simulink model "Joey_Control"  (R2022b)
settings: Solver=VariableStepAuto  StartTime=0.0  StopTime=3  RelTol=1e-3
libraries: simulink_extras x4
settings Model: Creator=khemwutapornpipatsakul  LastModifiedBy=khemwutapornpipatsakul

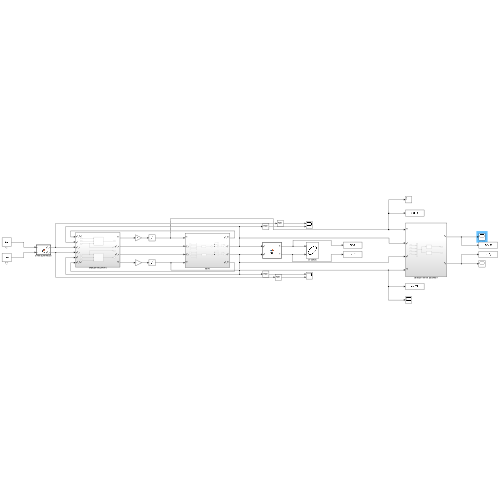
[thumbnail: Simulink's stored preview of the top-level diagram]
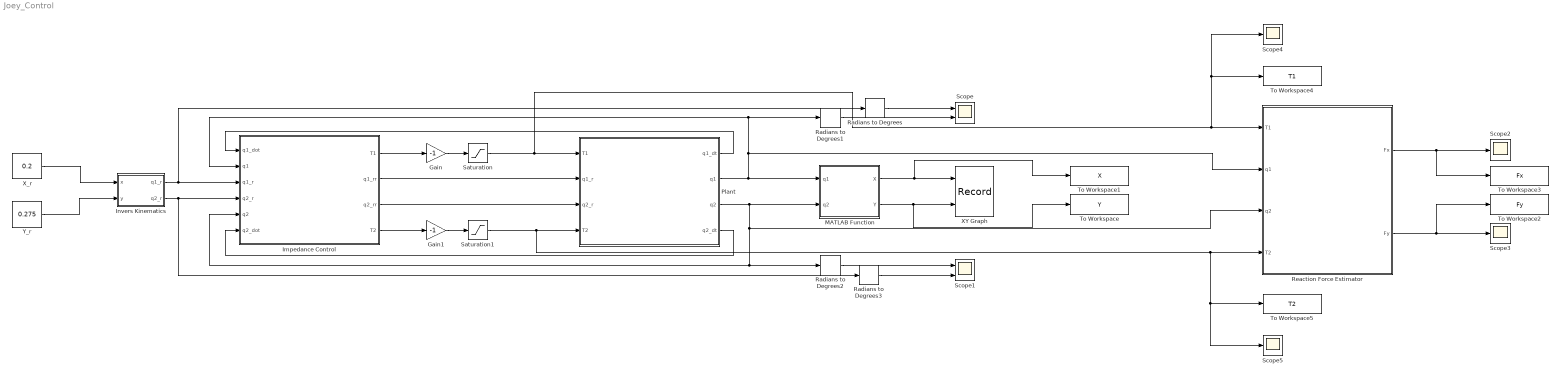
== system Joey_Control ==
  Gain : Gain  Gain=-1
  Gain1 : Gain  Gain=-1
  Impedance Control : Subsystem
  Invers Kinematics : MATLAB Function  TreatAsAtomicUnit=on
  MATLAB Function : MATLAB Function  TreatAsAtomicUnit=on
  Plant : Subsystem
  Radians to Degrees{,1..3} (4 alike) : simulink_extras/Transformations/Radians to Degrees
  Reaction Force Estimator : Subsystem
  Saturation : Saturate  UpperLimit=2  LowerLimit=-2
  Saturation1 : Saturate  UpperLimit=2  LowerLimit=-2
  Scope : Scope  NumInputPorts=2
  Scope1 : Scope  NumInputPorts=2
  Scope{2..5} (4 alike) : Scope
  To Workspace : ToWorkspace  VariableName=Y  SaveFormat=Timeseries  SampleTime=-1
  To Workspace1 : ToWorkspace  VariableName=X  SaveFormat=Timeseries  SampleTime=-1
  To Workspace2 : ToWorkspace  VariableName=Fy  SaveFormat=Timeseries  SampleTime=-1
  To Workspace3 : ToWorkspace  VariableName=Fx  SaveFormat=Timeseries  SampleTime=-1
  To Workspace4 : ToWorkspace  VariableName=T1  SaveFormat=Timeseries  SampleTime=-1
  To Workspace5 : ToWorkspace  VariableName=T2  SaveFormat=Timeseries  SampleTime=-1
  XY Graph : Record  FileSettingsInternal="{\"entries\":[{\"content\":{\"excelSettings\":{\"content\":{},\"type\":\"Streamout.ExcelSettings\"}},\"type\":\"Streamout.FileSettingStorage\",\"uuid\":\"b0abfdfa-5850-41cf-a1e0-bf550fd7b288\"}],\"packageUris\":[\"http://schema.mathworks.com/mf0/streamout_blocks/R2020a\"],\"version\":\"1.0\"}"  Layout=[1 1]  SignalsInternal="{\"entries\":[{\"content\":{\"signals\":[{\"content\":{\"blockPath\":[\"Joey_Control/XY Graph\"],\"channel\":[],\"dimensions\":[1],\"domain\":\"Joey_Control/XY Graph\",\"lineColor\":\"#a2142f\",\"plots\":[1],\"port\":1,\"sid\":[\"\"],\"signalID\":89,\"signalName\":\"MATLAB Function:1\"},\"type\":\"RecordBlkView.Signal\",\"uuid\":\"3823b3a6-9026-4afb-b3d4-39afb66ecd92\"},{\"content\":{\"blockPath\":[\"Joey_Control/XY Graph\"],\"channel\":[],\"dimensions\":[1],\"domain\":\"Joey_Control/XY Graph\",\"lineColor\":\"#139fff\",\"plots\":[1],\"port\":2,\"sid\":[\"\"],\"signalID\":93,\"signalName\":\"MATLAB Function:2\"},\"type\":\"RecordBlkView.Signal\",\"uuid\":\"4a1dff9e-01f1-4793-a448-94da4f18f44a\"}]},\"type\":\"RecordBlkView.InputSignals\",\"uuid\":\"29e68c19-1a98-4a03-81c8-2dcea01dd2a8\"}],\"packageUris\":[\"http://schema.mathworks.com/mf0/streamout_blocks/R2020a\"],\"version\":\"1.0\"}"  VisualizationBindings="{\"xyplotplugin\":{\"info\":[{\"series\":[{\"bindingParametersList\":[{\"parameter\":\"X-Axis\",\"signalID\":89,\"signalName\":\"MATLAB Function:1\"},{\"parameter\":\"Y-Axis\",\"signalID\":93,\"signalName\":\"MATLAB Function:2\"}],\"seriesID\":54391}],\"subplotID\":1}]}}"  CompatibilityTag=XY
  X_r : Constant  Value=0.2  SampleTime=0.01
  Y_r : Constant  Value=0.275  SampleTime=0.01
  wires:
  X_r/1 -> Invers Kinematics/1(x)
  Y_r/1 -> Invers Kinematics/2(y)
  Invers Kinematics/1(q1_r) -> Radians to Degrees/1, Impedance Control/3(q1_r)
  Invers Kinematics/2(q2_r) -> Radians to Degrees3/1, Impedance Control/4(q2_r)
  Impedance Control/1(T1) -> Gain/1
  Impedance Control/4(T2) -> Gain1/1
  Saturation/1 -> Scope4/1, To Workspace4/1, Reaction Force Estimator/1(T1), Plant/1(T1)
  Saturation1/1 -> Plant/4(T2), Scope5/1, To Workspace5/1, Reaction Force Estimator/4(T2)
  Impedance Control/2(q1_rr) -> Plant/2(q1_r)
  Impedance Control/3(q2_rr) -> Plant/3(q2_r)
  Plant/4(q2_dt) -> Impedance Control/6(q2_dot)
  Plant/1(q1_dt) -> Impedance Control/1(q1_dot)
  Plant/2(q1) -> MATLAB Function/1(q1), Impedance Control/2(q1), Radians to Degrees1/1, Reaction Force Estimator/2(q1)
  Plant/3(q2) -> Impedance Control/5(q2), Radians to Degrees2/1, Reaction Force Estimator/3(q2), MATLAB Function/2(q2)
  Gain/1 -> Saturation/1
  Gain1/1 -> Saturation1/1
  Reaction Force Estimator/1(Fx) -> To Workspace3/1, Scope2/1
  Reaction Force Estimator/2(Fy) -> To Workspace2/1, Scope3/1
  MATLAB Function/1(X) -> XY Graph/1, To Workspace1/1
  MATLAB Function/2(Y) -> XY Graph/2, To Workspace/1
  Radians to Degrees/1 -> Scope/1
  Radians to Degrees1/1 -> Scope/2
  Radians to Degrees2/1 -> Scope1/1
  Radians to Degrees3/1 -> Scope1/2

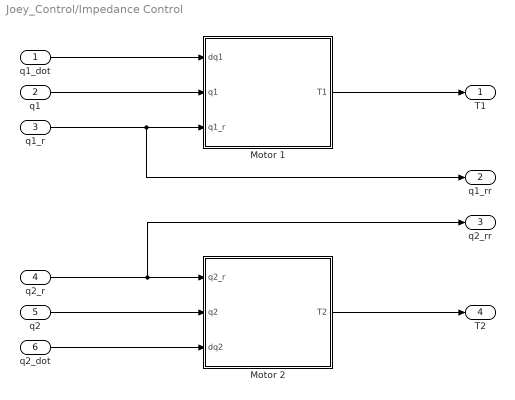
== system Joey_Control/Impedance Control ==
  q1_dot : Inport
  q1 : Inport  Port=2
  q1_r : Inport  Port=3
  q2_r : Inport  Port=4
  q2 : Inport  Port=5
  q2_dot : Inport  Port=6
  Motor 1 : MATLAB Function  TreatAsAtomicUnit=on
  Motor 2 : MATLAB Function  TreatAsAtomicUnit=on
  T1 : Outport
  q1_rr : Outport  Port=2
  q2_rr : Outport  Port=3
  T2 : Outport  Port=4
  wires:
  q1_dot/1 -> Motor 1/1(dq1)
  q1/1 -> Motor 1/2(q1)
  q1_r/1 -> q1_rr/1, Motor 1/3(q1_r)
  Motor 1/1(T1) -> T1/1
  q2_r/1 -> q2_rr/1, Motor 2/1(q2_r)
  q2/1 -> Motor 2/2(q2)
  q2_dot/1 -> Motor 2/3(dq2)
  Motor 2/1(T2) -> T2/1

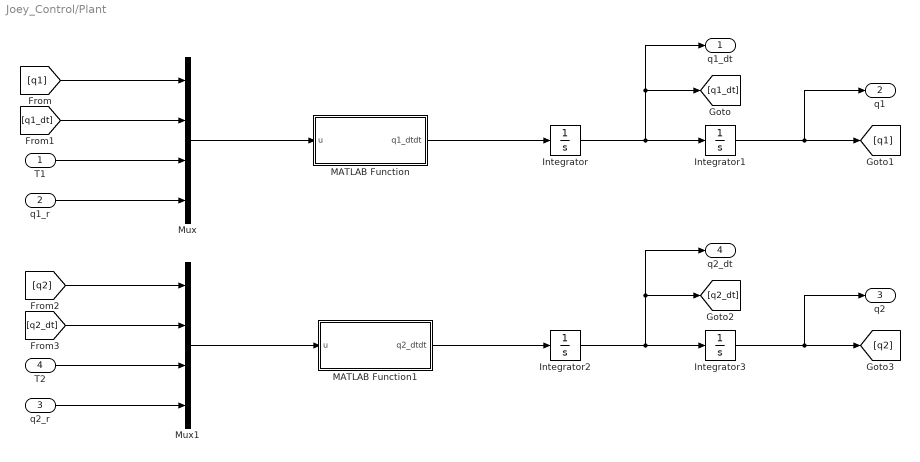
== system Joey_Control/Plant ==
  T1 : Inport
  q1_r : Inport  Port=2
  q2_r : Inport  Port=3
  T2 : Inport  Port=4
  Integrator{,1..3} (4 alike) : Integrator
  MATLAB Function : MATLAB Function  TreatAsAtomicUnit=on
  MATLAB Function1 : MATLAB Function  TreatAsAtomicUnit=on
  Mux : Mux
  Mux1 : Mux
  q1_dt : Outport
  q1 : Outport  Port=2
  q2 : Outport  Port=3
  q2_dt : Outport  Port=4
  wires:
  [q1_dt] -> Mux/2
  T1/1 -> Mux/3
  q1_r/1 -> Mux/4
  [q1] -> Mux/1
  Mux/1 -> MATLAB Function/1(u)
  Mux1/1 -> MATLAB Function1/1(u)
  MATLAB Function/1(q1_dtdt) -> Integrator/1
  Integrator/1 -> q1_dt/1, [q1_dt], Integrator1/1
  Integrator1/1 -> q1/1, [q1]
  MATLAB Function1/1(q2_dtdt) -> Integrator2/1
  Integrator3/1 -> q2/1, [q2]
  Integrator2/1 -> q2_dt/1, [q2_dt], Integrator3/1
  [q2_dt] -> Mux1/2
  [q2] -> Mux1/1
  T2/1 -> Mux1/3
  q2_r/1 -> Mux1/4

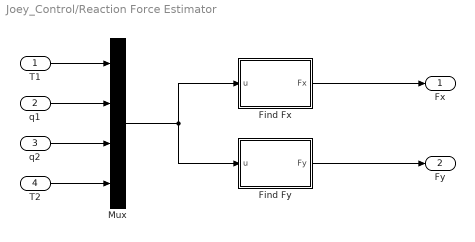
== system Joey_Control/Reaction Force Estimator ==
  T1 : Inport
  q1 : Inport  Port=2
  q2 : Inport  Port=3
  T2 : Inport  Port=4
  Find Fx : MATLAB Function  TreatAsAtomicUnit=on
  Find Fy : MATLAB Function  TreatAsAtomicUnit=on
  Mux : Mux
  Fx : Outport
  Fy : Outport  Port=2
  wires:
  T1/1 -> Mux/1
  q1/1 -> Mux/2
  q2/1 -> Mux/3
  T2/1 -> Mux/4
  Mux/1 -> Find Fy/1(u), Find Fx/1(u)
  Find Fx/1(Fx) -> Fx/1
  Find Fy/1(Fy) -> Fy/1

== matlab function Joey_Control/Invers Kinematics ==
  data: x input; q1_r output; y input; q2_r output
function [q1_r,q2_r] = fcn(x,y)

q1_r = atan((x.*2.2e+4-sqrt(x.^2.*y.^2.*-3.2e+9+x.^2.*4.2632e+8-x.^4.*1.6e+9+y.^2.*4.2632e+8-y.^4.*1.6e+9-5.19841e+5))./(y.*2.2e+4+x.^2.*4.0e+4+y.^2.*4.0e+4+7.21e+2)).*2.0;
q2_r = atan((y.*1.92e+4-sqrt(-(x.^2.*4.0e+4+y.^2.*4.0e+4-4.9e+1).*(x.^2.*4.0e+4+y.^2.*4.0e+4-1.0609e+4)))./(x.*1.92e+4+x.^2.*4.0e+4+y.^2.*4.0e+4-7.21e+2)).*-2.0;

end

== matlab function Joey_Control/Impedance Control/Motor 2 ==
  data: q2_r input; q2 input; dq2 input; T2 output
function T2 = fcn(q2_r,q2,dq2)

    T2 = 1*dq2 + 5*(q2-q2_r);

end

== matlab function Joey_Control/Plant/MATLAB Function ==
  data: u input; q1_dtdt output
function q1_dtdt = fcn(u)

    q1_dtdt = (u(3) - 0.05*(u(2)) - 0*(u(1)-u(4)))/0.043;
%     q1_dtdt = 0

end

== matlab function Joey_Control/Plant/MATLAB Function1 ==
  data: u input; q2_dtdt output
function q2_dtdt = fcn(u)

    q2_dtdt = (u(3) - 0.5*(u(2)) - 0.05*(u(1)-u(4)))/0.234;
%     q2_dtdt = 0

end

== matlab function Joey_Control/Reaction Force Estimator/Find Fx ==
  data: u input; Fx output
function Fx = fcn(u)

Fx = ((u(1).*cos(u(2)-u(3)+pi.*(2.0./5.0)).*cos(u(3)).*(-6.0./2.5e+1)+u(4).*sin(u(2)).^2.*sin(u(3)+pi./1.0e+1).*(1.1e+1./4.0e+1)+u(4).*cos(u(2)).*cos(u(3)+pi./1.0e+1).*sin(u(2)).*(1.1e+1./4.0e+1)).*(5.0e+2./3.3e+1))./(cos(u(2)-u(3)+pi.*(2.0./5.0)).*(cos(u(2)).*cos(u(3))+sin(u(2)).*sin(u(3))));


end

== matlab function Joey_Control/Reaction Force Estimator/Find Fy ==
  data: u input; Fy output
function Fy= fcn(u)

Fy = ((u(1).*cos(u(2)-u(3)+pi.*(2.0./5.0)).*sin(u(3)).*(6.0./2.5e+1)+u(4).*cos(u(2)).^2.*cos(u(3)+pi./1.0e+1).*(1.1e+1./4.0e+1)+u(4).*cos(u(2)).*sin(u(2)).*sin(u(3)+pi./1.0e+1).*(1.1e+1./4.0e+1)).*(5.0e+2./3.3e+1))./(cos(u(2)-u(3)+pi.*(2.0./5.0)).*(cos(u(2)).*cos(u(3))+sin(u(2)).*sin(u(3))));

end

== matlab function Joey_Control/MATLAB Function ==
  data: q1 input; X output; q2 input; Y output
function [X,Y] = fcn(q1,q2)
    
    X = 0.275.*sin(q1)+0.24.*cos(q2)
    Y = 0.275.*cos(q1)-0.24.*sin(q2)
end

== matlab function Joey_Control/Impedance Control/Motor 1 ==
  data: dq1 input; q1 input; q1_r input; T1 output
function T1 = fcn(dq1,q1,q1_r)

    T1 = 1*dq1 + 5*(q1-q1_r);

end
